simulink model "EReg_v2"  (R2025b)
settings: Solver=FixedStepDiscrete  StartTime=0.0  StopTime=Sim_Duration  FixedStep=Ts_sim  RelTol=1e-3
undefined symbols (not defined in the file): A_3, backlash_init, Cd_3, DiscIntNeverNeededParam, gamma_N2, K_v_4, Kv_1_max, m_1_0, m_2_0, m_3_0, Pst, R_N2, rho_1_0, rho_L, rhost, T_0_N2, Ts_ctrl, Ts_sim, Tst, V_1, V_2
settings Model: Creator=ethan  LastModifiedBy=ethan
settings DebuggingCC: AlgebraicLoopMsg=error

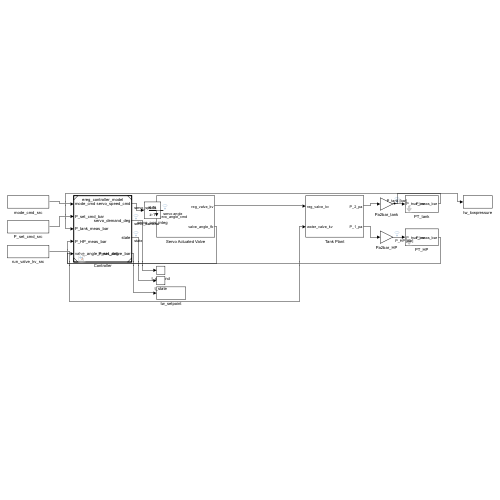
[thumbnail: Simulink's stored preview of the top-level diagram]
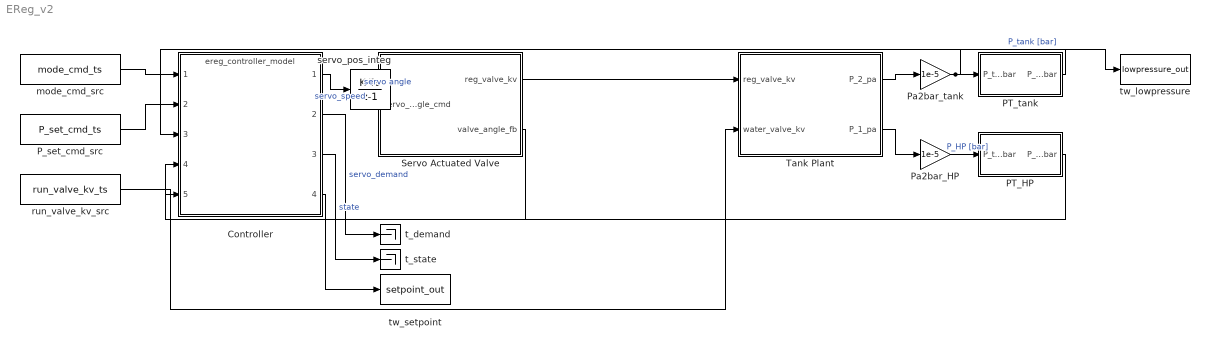
== system EReg_v2 ==
  Controller : ModelReference  ModelNameDialog=ereg_controller_model  SimulationMode=Normal  ModelReferenceVersion=1.1
  PT_HP : Subsystem  mask{Ts_pt=0, noise_std_bar=0, quant_lsb_bar=0, seed=0}
      mask prompts: Ts_pt "PT sample time [s]"; noise_std_bar "Noise std [bar]"; quant_lsb_bar "Quantization LSB [bar]"; seed "Noise seed"
      mask help:
      | Pressure transducer placeholder (pure passthrough).
      | Upgrade recipe: inside, insert ZOH (Ts_pt) -> add Random Number (seed, noise_std_bar) -> Quantizer (quant_lsb_bar). Mask params are declared but unused until then.
  PT_tank : Subsystem  mask{Ts_pt=0, noise_std_bar=0, quant_lsb_bar=0, seed=0}
      mask prompts: Ts_pt "PT sample time [s]"; noise_std_bar "Noise std [bar]"; quant_lsb_bar "Quantization LSB [bar]"; seed "Noise seed"
      mask help:
      | Pressure transducer placeholder (pure passthrough).
      | Upgrade recipe: inside, insert ZOH (Ts_pt) -> add Random Number (seed, noise_std_bar) -> Quantizer (quant_lsb_bar). Mask params are declared but unused until then.
  P_set_cmd_src : FromWorkspace  VariableName=P_set_cmd_ts  SampleTime=Ts_sim  ZeroCross=off  OutputAfterFinalValue=Holding final value
  Pa2bar_HP : Gain  Gain=1e-5
  Pa2bar_tank : Gain  Gain=1e-5
  Servo Actuated Valve : Subsystem
  Tank Plant : Subsystem
  mode_cmd_src : FromWorkspace  VariableName=mode_cmd_ts  SampleTime=Ts_sim  Interpolate=off  ZeroCross=off  OutputAfterFinalValue=Holding final value
  run_valve_kv_src : FromWorkspace  VariableName=run_valve_kv_ts  SampleTime=Ts_sim  ZeroCross=off  OutputAfterFinalValue=Holding final value
  servo_pos_integ : DiscreteIntegrator  SampleTime=Ts_ctrl  ICPrevOutput=DiscIntNeverNeededParam  ICPrevScaledInput=DiscIntNeverNeededParam
  t_demand : Terminator
  t_state : Terminator
  tw_lowpressure : ToWorkspace  VariableName=lowpressure_out  SaveFormat=Timeseries  SampleTime=-1
  tw_setpoint : ToWorkspace  VariableName=setpoint_out  SaveFormat=Timeseries  SampleTime=-1
  wires:
  mode_cmd_src/1 -> Controller/1
  P_set_cmd_src/1 -> Controller/2
  Controller/1 -> servo_pos_integ/1  "servo_speed"
  servo_pos_integ/1 -> Servo Actuated Valve/1(servo_angle_cmd)  "servo angle"
  Controller/2 -> t_demand/1  "servo_demand"
  Controller/3 -> t_state/1  "state"
  Controller/4 -> tw_setpoint/1
  Servo Actuated Valve/1(reg_valve_kv) -> Tank Plant/1(reg_valve_kv)
  run_valve_kv_src/1 -> Tank Plant/2(water_valve_kv)
  Tank Plant/1(P_2_pa) -> Pa2bar_tank/1
  Pa2bar_tank/1 -> PT_tank/1(P_true_bar), tw_lowpressure/1  "P_tank [bar]"
  PT_tank/1(P_meas_bar) -> Controller/3
  Tank Plant/2(P_1_pa) -> Pa2bar_HP/1
  Pa2bar_HP/1 -> PT_HP/1(P_true_bar)  "P_HP [bar]"
  PT_HP/1(P_meas_bar) -> Controller/4
  Servo Actuated Valve/2(valve_angle_fb) -> Controller/5

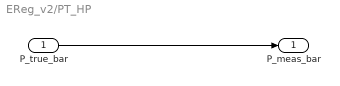
== system EReg_v2/PT_HP ==
  P_true_bar : Inport
  P_meas_bar : Outport
  wires:
  P_true_bar/1 -> P_meas_bar/1

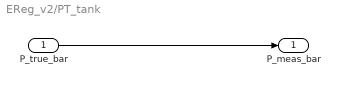
== system EReg_v2/PT_tank ==
  P_true_bar : Inport
  P_meas_bar : Outport
  wires:
  P_true_bar/1 -> P_meas_bar/1

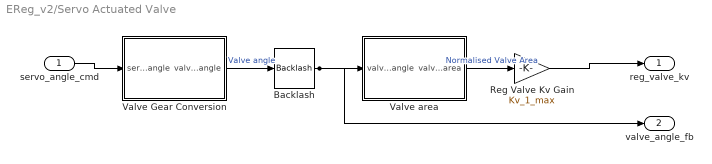
== system EReg_v2/Servo Actuated Valve ==
  servo_angle_cmd : Inport
  Backlash : Backlash  BacklashWidth=backlash_width  InitialOutput=backlash_init
  Reg Valve Kv Gain : Gain  Gain=Kv_1_max
  Valve Gear Conversion : MATLAB Function  TreatAsAtomicUnit=on
  Valve area : MATLAB Function  TreatAsAtomicUnit=on
  reg_valve_kv : Outport
  valve_angle_fb : Outport  Port=2
  wires:
  servo_angle_cmd/1 -> Valve Gear Conversion/1(servo_angle)
  Valve Gear Conversion/1(valve_angle) -> Backlash/1  "Valve angle"
  Backlash/1 -> Valve area/1(valve_angle), valve_angle_fb/1
  Valve area/1(valve_area) -> Reg Valve Kv Gain/1  "Normalised Valve Area"
  Reg Valve Kv Gain/1 -> reg_valve_kv/1

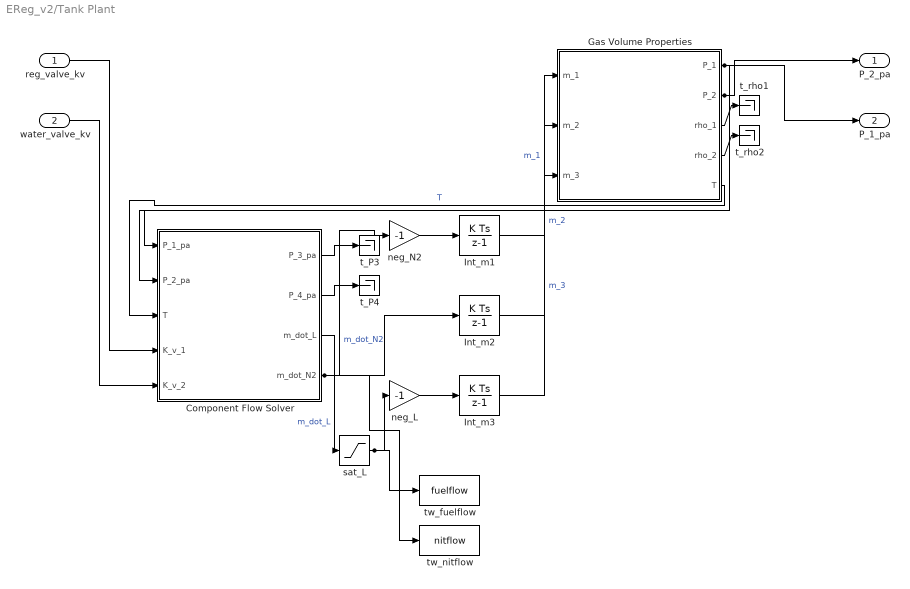
== system EReg_v2/Tank Plant ==
  reg_valve_kv : Inport
  water_valve_kv : Inport  Port=2
  Component Flow Solver : MATLAB Function  TreatAsAtomicUnit=on
  Gas Volume Properties : MATLAB Function  TreatAsAtomicUnit=on
  Int_m1 : DiscreteIntegrator  InitialCondition=m_1_0  SampleTime=Ts_sim  ICPrevOutput=DiscIntNeverNeededParam  ICPrevScaledInput=DiscIntNeverNeededParam
  Int_m2 : DiscreteIntegrator  InitialCondition=m_2_0  SampleTime=Ts_sim  ICPrevOutput=DiscIntNeverNeededParam  ICPrevScaledInput=DiscIntNeverNeededParam
  Int_m3 : DiscreteIntegrator  InitialCondition=m_3_0  SampleTime=Ts_sim  ICPrevOutput=DiscIntNeverNeededParam  ICPrevScaledInput=DiscIntNeverNeededParam
  neg_L : Gain  Gain=-1
  neg_N2 : Gain  Gain=-1
  sat_L : Saturate  UpperLimit=inf  LowerLimit=0
  t_P3 : Terminator
  t_P4 : Terminator
  t_rho1 : Terminator
  t_rho2 : Terminator
  tw_fuelflow : ToWorkspace  VariableName=fuelflow  SaveFormat=Timeseries  SampleTime=-1
  tw_nitflow : ToWorkspace  VariableName=nitflow  SaveFormat=Timeseries  SampleTime=-1
  P_2_pa : Outport
  P_1_pa : Outport  Port=2
  wires:
  Gas Volume Properties/1(P_1) -> Component Flow Solver/1(P_1_pa), P_1_pa/1
  Gas Volume Properties/2(P_2) -> Component Flow Solver/2(P_2_pa), P_2_pa/1
  Gas Volume Properties/5(T) -> Component Flow Solver/3(T)  "T"
  Gas Volume Properties/3(rho_1) -> t_rho1/1
  Gas Volume Properties/4(rho_2) -> t_rho2/1
  reg_valve_kv/1 -> Component Flow Solver/4(K_v_1)
  water_valve_kv/1 -> Component Flow Solver/5(K_v_2)
  Component Flow Solver/1(P_3_pa) -> t_P3/1
  Component Flow Solver/2(P_4_pa) -> t_P4/1
  Component Flow Solver/3(m_dot_L) -> sat_L/1  "m_dot_L"
  sat_L/1 -> neg_L/1, tw_fuelflow/1
  neg_L/1 -> Int_m3/1
  Component Flow Solver/4(m_dot_N2) -> neg_N2/1, Int_m2/1, tw_nitflow/1  "m_dot_N2"
  neg_N2/1 -> Int_m1/1
  Int_m1/1 -> Gas Volume Properties/1(m_1)  "m_1"
  Int_m2/1 -> Gas Volume Properties/2(m_2)  "m_2"
  Int_m3/1 -> Gas Volume Properties/3(m_3)  "m_3"

== matlab function EReg_v2/Tank Plant/Component Flow Solver ==
  data: P_1_pa input; P_3_pa output; P_2_pa input; T input; K_v_1 input; K_v_2 input; P_4_pa output; m_dot_L output; m_dot_N2 output; Cd_3 parameter; K_v_4 parameter; rho_L parameter; R_N2 parameter; Tst parameter; rhost parameter; A_3 parameter; Pst parameter
function [P_3_pa, P_4_pa, m_dot_L, m_dot_N2] = fcn(P_1_pa, P_2_pa, T, K_v_1, K_v_2, Cd_3, K_v_4, rho_L, R_N2, Tst, rhost, A_3, Pst)
%#codegen

% This function solves for the intermediate pressures and mass flows in a
% fluid system. It replaces a non-codegen-compatible 'fsolve' call with
% two independent 1D Newton-Raphson solvers.

% --- Solver Parameters ---
MAX_ITER = 50;  % Maximum iterations for Newton's method
TOLERANCE = 1e-7; % Convergence tolerance
h = 1e-6;       % Step size for numerical derivative
P_atm_pa = 101325;
% --- Input Conversions ---
% Convert input pressures from Pascals (pa) to bar for K_v calcs
P_1 = P_1_pa * 1e-5;
P_2 = P_2_pa * 1e-5;
% Note: P_atm_pa is passed directly to calc_m_dot_b, which expects Pascals

% --- Problem Setup ---
% Calculate Specific Gravity for liquid flow
SG = rho_L / 1000.0;

% --- 1. Solve for Liquid-Side Pressure P_3 ---
% We need to find P_3 (in bar) such that: liquid_error(P_3) = 0
% where liquid_error = calc_m_dot_a(P_3) - calc_m_dot_b(P_3)

% Define the error function for the liquid side
% All parameters are passed anonymously
liquid_error_fun = @(p3) (calc_m_dot_a(p3, P_2, K_v_2, rho_L, SG) - ...
                          calc_m_dot_b(p3, Cd_3, A_3, rho_L, P_atm_pa));

% Initial guess for P_3 (in bar)
x0_P3 = 1.0; 

% Call the Newton solver
P_3_bar = newton_solver(liquid_error_fun, x0_P3, MAX_ITER, TOLERANCE, h);

% --- 2. Solve for Gas-Side Pressure P_4 ---
% We need to find P_4 (in bar) such that: gas_error(P_4) = 0
% where gas_error = calc_m_dot_c(P_4) - calc_m_dot_d(P_4)

% Define the error function for the gas side
gas_error_fun = @(p4) (calc_m_dot_c(p4, P_1, K_v_1, rhost, T, Pst, R_N2, Tst) - ...
                       calc_m_dot_d(p4, P_2, K_v_4, rhost, T, Pst, R_N2, Tst));
                       
% Initial guess for P_4 (in bar)
x0_P4 = 1.0; 

% Call the Newton solver
P_4_bar = newton_solver(gas_error_fun, x0_P4, MAX_ITER, TOLERANCE, h);

% --- 3. Calculate Final Outputs ---
% Convert pressures back to Pascals
P_3_pa = P_3_bar * 1e5;
P_4_pa = P_4_bar * 1e5;

% Calculate the final mass flow rates using the solved pressures
m_dot_L  = calc_m_dot_a(P_3_bar, P_2, K_v_2, rho_L, SG);
m_dot_N2 = calc_m_dot_c(P_4_bar, P_1, K_v_1, rhost, T, Pst, R_N2, Tst);

end

% =========================================================================
% --- NESTED HELPER FUNCTIONS (CODEGEN-COMPATIBLE) ---
% =========================================================================

function x_root = newton_solver(fun, x0, max_iter, tol, h)
% A simple 1D Newton-Raphson solver using a numerical derivative.
% It finds x such that fun(x) = 0.
    
    x_root = x0;
    for i = 1:max_iter
        % Calculate function value at current point
        f_val = fun(x_root);
        
        % Check for convergence
        if abs(f_val) < tol
            return; % Solution found
        end
        
        % Calculate function value at a small step h away
        f_val_h = fun(x_root + h);
        
        % Calculate numerical derivative (Jacobian)
        f_deriv = (f_val_h - f_val) / h;
        
        % Check for division by zero (flat gradient)
        if abs(f_deriv) < 1e-10
            % Cannot converge, return last best guess
            return;
        end
        
        % Newton's step
        x_new = x_root - f_val / f_deriv;
        
        % Check for step convergence
        if abs(x_new - x_root) < tol
            x_root = x_new;
            return; % Solution found
        end
        
        x_root = x_new;
    end
    % If loop finishes, max iterations were reached. Return last value.
end


function m_dot_a = calc_m_dot_a(P_3, P_2, K_v_2, rho_L, SG)
% Water Control Valve (m_dot_a)
% All pressures in bar
    delta_P = P_2 - P_3;
    % Use sign(delta_P) to handle potential flow reversal safely
    Q = K_v_2 * (delta_P / SG) / sqrt(abs(delta_P / SG) + 1e-9); 
    m_dot_a = Q * rho_L * (1/3600); % Convert standard flow rate to mass flow rate
end


function m_dot_b = calc_m_dot_b(P_3_bar, Cd_3, A_3, rho_L, P_atm_pa)
% Water Orifice (m_dot_b)
% P_3_bar is in bar, P_atm_pa is in Pascals
    
    % Convert P_3 from bar to Pascals for this equation
    P_3_pa = P_3_bar * 1e5;
    delta_P_pa = P_3_pa - P_atm_pa;
    
    % This formulation from your original code correctly handles flow
    % direction using sign(delta_P) * sqrt(abs(delta_P))
    m_dot_b = Cd_3 * A_3 * 2 * rho_L * delta_P_pa / sqrt(abs(2 * rho_L * delta_P_pa) + 1e-9);
end


function m_dot_c = calc_m_dot_c(P_4, P_1, K_v_1, rhost, T, Pst, R_N2, Tst)
% Regulator Valve (m_dot_c)
% All pressures in bar
    Q_N = 0.0;
    if (P_4 >= 0.528 * P_1)
        % Non-choked flow
        arg = (P_1 - P_4) * P_4 / (rhost * T);
        Q_N = K_v_1 * 514 * arg / sqrt(abs(arg) + 1e-9);
    else
        % Choked flow
        Q_N = K_v_1 * 257 * P_1 / sqrt(abs(rhost * T) + 1e-9);
    end
    m_dot_c = Q_N * (Pst / (R_N2 * Tst)) * (1/3600); % Convert standard flow rate to mass flow rate
end


function m_dot_d = calc_m_dot_d(P_4, P_2, K_v_4, rhost, T, Pst, R_N2, Tst)
% Check Valve (m_dot_d)
% All pressures in bar
    Q_N = 0.0;
    if (P_2 >= 0.528 * P_4)
        % Non-choked flow
        arg = (P_4 - P_2) * P_2 / (rhost * T);
        Q_N = K_v_4 * 514 * arg / sqrt(abs(arg) + 1e-9);
    else
        % Choked flow
        Q_N = K_v_4 * 257 * P_4 / sqrt(abs(rhost * T) + 1e-9);
    end
    m_dot_d = Q_N * (Pst / (R_N2 * Tst)) * (1/3600); % Convert standard flow rate to mass flow rate
end

== matlab function EReg_v2/Tank Plant/Gas Volume Properties ==
  data: m_1 input; P_1 output; m_2 input; m_3 input; P_2 output; rho_1 output; rho_2 output; T output; V_1 parameter; V_2 parameter; T_0_N2 parameter; rho_1_0 parameter; gamma_N2 parameter; R_N2 parameter; rho_L parameter
function [P_1, P_2, rho_1, rho_2, T]= fcn(m_1, m_2, m_3, V_1, V_2, T_0_N2, rho_1_0, gamma_N2, R_N2, rho_L)

rho_1 = m_1/V_1; %Find the HP tank gas density
rho_2 = m_2/(V_2 - m_3/rho_L); %Find the ullage gas density
T = T_0_N2*(rho_1/rho_1_0)^(gamma_N2 - 1); %Find the ullage gas temperature (assumiong adiabatic expansion)
P_1 = rho_1*R_N2*T; %Find the HP gas pressure
P_2 = rho_2*R_N2*T; %Find the ullage gas pressure (Tank pressure)

== matlab function EReg_v2/Servo Actuated Valve/Valve Gear Conversion ==
  data: servo_angle input; valve_angle output
function valve_angle = fcn(servo_angle)

valve_angle = servo_angle/1.7; % check gear ratio with oscar
%valve_angle = servo_angle;

== matlab function EReg_v2/Servo Actuated Valve/Valve area ==
  data: valve_angle input; valve_area output
function valve_area = fcn(valve_angle)
%     % BUG RECREATION: hardware has angle convention inverted vs sim
%     % Sim convention was: 0°=closed, 90°=open
%     % Hardware reality:   0°=open,   90°=closed
%     % Equivalent: feed (90 - valve_angle) through the same polynomial
%     inverted_angle = 90 - valve_angle;
%     inverted_angle = inverted_angle - 5;  % keep the same deadband
%     if inverted_angle < 0
%         valve_area = 0;
%     else
%         valve_area = 1.1*((5*10^-6)*inverted_angle^3 - 0.0006*inverted_angle^2 + 0.0278*inverted_angle);
%     end
% end

valve_angle = valve_angle - 5; %Account for first part of rotation where valve doesn't open at all
if valve_angle < 0
    valve_area = 0;
else
    valve_area = 1.1*((5*10^-6)*valve_angle^3 - 0.0006*valve_angle^2 + 0.0278*valve_angle); %calculate normalised valve area
end
